simulink model "SignalToNoiseDSKC6713"  (Simulink 6.5)
settings: Solver=FixedStepDiscrete  StartTime=0.0  StopTime=inf  RelTol=1e-3
PreLoadFcn:
  | load dspwlets;
PostLoadFcn:
  | c6000demoscallback
undefined symbols (not defined in the file or in its folder): bit, D, fdesignblkfcn, gcbh
libraries: dspsigops x11, c6713dsklib x4, dspstat3 x3, simulink x1, dspsigattribs x1, dspmathops x1, c6000tgtpreflib x1, dspbioslib x1
CloseFcn:
  | clear fs hid hir lod lor noisdopp ts;
settings Model: RequirementInfo=9  Creator=don  LastModifiedBy=Administrator  CovMetricSettings=d  ExtModeTrigMode=oneshot  ExtModeArmWhenConnect=off  ProdHWDeviceType=TI C6000
settings SolverCC: PositivePriorityOrder=on
settings DataIOCC: LimitDataPoints=off  SaveOutput=off  SaveTime=off  SignalLoggingName=sigsOut
settings OptimizationCC: BlockReduction=off  BooleanDataType=off  InlineParams=on  InlineInvariantSignals=on  RollThreshold=2  OptimizeModelRefInitCode=on  LifeSpan=1  BufferReusableBoundary=off
settings DebuggingCC: CheckExecutionContextPreStartOutputMsg=on  CheckExecutionContextRuntimeOutputMsg=on  SolverPrmCheckMsg=none  InheritedTsInSrcMsg=none  MultiTaskDSMMsg=warning  MultiTaskCondExecSysMsg=none  IntegerOverflowMsg=none  StrictBusMsg=None
settings HardwareCC: ProdBitPerLong=40  ProdIntDivRoundTo=Zero  ProdEndianess=LittleEndian  ProdHWDeviceType=TI C6000  TargetHWDeviceType=32-bit Generic
settings ModelReferenceCC: UpdateModelReferenceTargets=IfOutOfDate
settings RTWCC: SystemTargetFile=ti_c6000_ert.tlc  GenCodeOnly=on  TemplateMakefile=ti_c6000_ert.tmf  ProcessScript=ti_c6000_ert_make_rtw_hook  IncludeERTFirstTime=on
settings CodeAppCC: IgnoreCustomStorageClasses=off  PrefixModelToSubsysFcnNames=off  CustomSymbolStrFcn=$F$N$M
settings C6000ERTTargetCC: TargetFcnLib=ansi_tfl_tmw.mat  GenFloatMathFcnCalls=ANSI_C  UtilityFuncGeneration=Auto  GenerateFullHeader=on  GenerateSampleERTMain=on  GenerateTestInterfaces=off  IsPILTarget=off  ModelReferenceCompliant=off  IncludeMdlTerminateFcn=on  CombineOutputUpdateFcns=on  SuppressErrorStatus=off  IncludeFileDelimiter=Auto  ERTCustomFileBanners=on  SupportAbsoluteTime=on  LogVarNameModifier=rt_  MatFileLogging=off  MultiInstanceERTCode=off  SupportNonFinite=on  SupportComplex=on  PurelyIntegerCode=off  SupportContinuousTime=on  SupportNonInlinedSFcns=on  EnableShiftOperators=on  ParenthesesLevel=Nominal  GenerateErtSFunction=off  GenerateASAP2=off  ExtMode=off  ExtModeTransport=0  ExtModeStaticAlloc=off  ExtModeStaticAllocSize=1000000  ExtModeTesting=off  ExtModeMexFile=ext_comm  InlinedParameterPlacement=NonHierarchical  TargetOS=BareBoardExample  MultiInstanceErrorCode=Error  RateGroupingCode=on  RootIOFormat=Individual arguments  RTWCAPISignals=off  RTWCAPIParams=off  RTWCAPIStates=off  ERTSrcFileBannerTemplate=ert_code_template.cgt  ERTHdrFileBannerTemplate=ert_code_template.cgt  ERTDataSrcFileTemplate=ert_code_template.cgt  ERTDataHdrFileTemplate=ert_code_template.cgt  ERTCustomFileTemplate=example_file_process.tlc  ModuleNamingRule=Unspecified  SignalDisplayLevel=10  ParamTuneLevel=10  GlobalDataDefinition=Auto  DataDefinitionFile=global.c  GlobalDataReference=Auto  DataReferenceFile=global.h  GRTInterface=off  EnableUserReplacementTypes=off  MemSecPackage=--- None ---  MemSecDataConstants=Default  MemSecDataIO=Default  MemSecDataInternal=Default  MemSecDataParameters=Default  MemSecFuncInitTerm=Default  MemSecFuncExecute=Default  exportCCSObj=on  ccsObjName=CCS_Obj  useDSPBIOS=on  ProfileGenCode=off  InlineDSPBlks=on  FPopt=off  memModel=Far_Aggregate  optLevel=Function(-o2)  CompilerVerbosity=Quiet  InterruptThreshOnC6x=off  SymbolicDebugOnC6x=off  RetainAsmFiles=off  RetainObjFiles=on  CreateMapFile=on  UserStackSize=8192  c6000BuildAction=Build_and_execute  OverrunAction=Notify_and_continue  OverrunNotificationMethod=Turn_on_LEDs

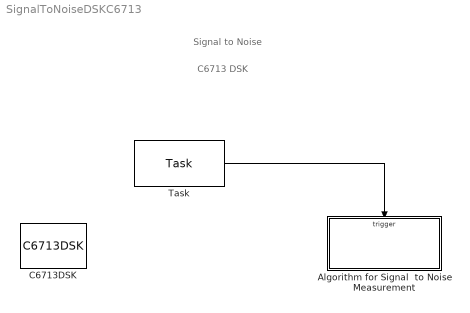
== system SignalToNoiseDSKC6713 ==
  note: C6713 DSK
  note: Signal to Noise
  Algorithm for Signal  to Noise Measurement : Subsystem  TreatAsAtomicUnit=on
  C6713DSK : c6000tgtpreflib/C6713DSK  Tag=C6000 TARGET PREFERENCES BLOCK  SystemSampleTime=-1
  Task : dspbioslib/Task  SystemSampleTime=-1  taskName=Task0  taskPriority=1  taskExecutionOrder=1  taskStackSize=16000  stackMemSegment=IRAM  monitorStackUse=off  taskYield=off  parentmanaget=on  tickres=1/1000  ticklen=32bits  taskTrigger=off
  wires:
  Task/1 -> Algorithm for Signal  to Noise Measurement/Trigger

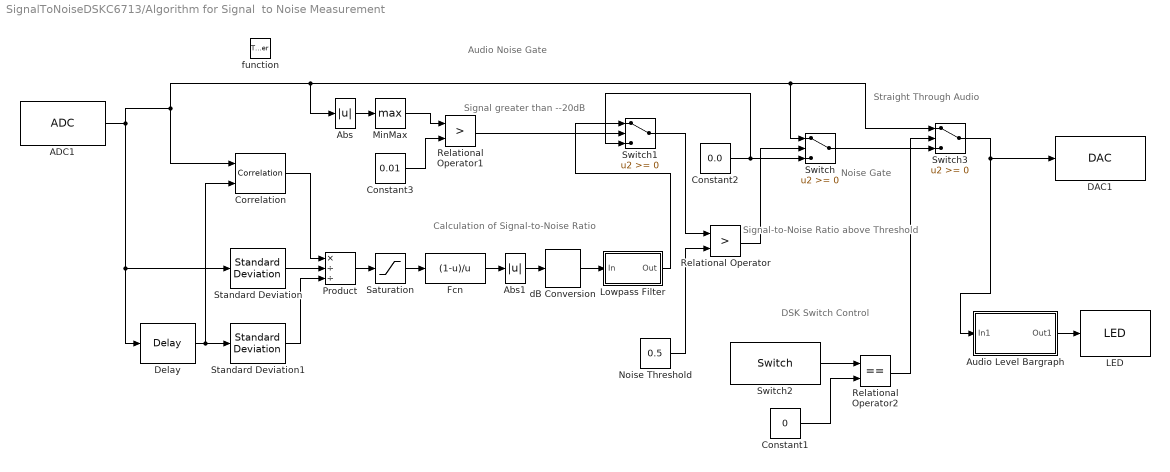
== system SignalToNoiseDSKC6713/Algorithm for Signal  to Noise Measurement ==
  note: Audio Noise Gate
  note: Calculation of Signal-to-Noise Ratio
  note: Signal greater
      |  than --20dB
  note: Straight
      | Through Audio
  note: Noise
      |  Gate
  note: DSK Switch Control
  note: Signal-to-Noise Ratio
      |  above Threshold
  function : TriggerPort  TriggerType=function-call
  ADC1 : c6713dsklib/ADC  ADCsource=Mic In  MicGain=on  Stereo=off  SampleRate=8 kHz  CodecDataFormat=16-bit  OutputDataType=Single  Scaling=Normalize  SourceGain=0.0  FrameSize=128  inheritSampleTime=on
  Abs : Abs  SampleTime=-1  SaturateOnIntegerOverflow=off
  Abs1 : Abs  SampleTime=-1  SaturateOnIntegerOverflow=off
  Audio Level Bargraph : Subsystem
  Constant1 : Constant  Value=0  OutDataType=sfix(16)  ConRadixGroup=Use specified scaling  OutScaling=2^0  SampleTime=inf  FramePeriod=inf
  Constant2 : Constant  Value=0.0  OutDataType=sfix(16)  ConRadixGroup=Use specified scaling  OutScaling=2^0  SampleTime=inf  FramePeriod=inf
  Constant3 : Constant  Value=0.01  OutDataType=sfix(16)  ConRadixGroup=Use specified scaling  OutScaling=2^0  SampleTime=inf  FramePeriod=inf
  Correlation : dspstat3/Correlation  DialogController=dspDDGCreate  DialogControllerArgs=DataTag0  domain=Time  roundingMode=Floor  overflowMode=off
  DAC1 : c6713dsklib/DAC  CodecDataFormat=16-bit  SampleRate=8 kHz  Scaling=Normalize  DacAtten=0.0  OverflowMode=Saturate
  Delay : dspsigops/Delay  dly_unit=Samples  delay=12  ic_detail=off  dif_ic_for_ch=off  dif_ic_for_dly=off  ic=0  reset_popup=None
  Fcn : Fcn  Expr=(1-u)/u
  LED : c6713dsklib/LED
  Lowpass Filter : Subsystem  DialogController=fdesignblkfcn  DialogControllerArgs=DataTag2  InitFcn=fdesignblkfcn(gcbh, {'InitFcn'});
      settings: CopyFcn=fdesignblkfcn(gcbh, {'CopyFcn'});
      mask Type: Lowpass Filter
      mask Description: Design a lowpass filter
      mask Help: helpview(mapfilelocation('dspblks'), 'dsplowpassfilter')
      mask Display: disp('Lowpass')
  MinMax : MinMax  Function=max
  "Noise Threshold " : Constant  Value=0.5  OutDataType=sfix(16)  ConRadixGroup=Use specified scaling  OutScaling=2^0  SampleTime=inf  FramePeriod=inf
  Product : Product  Inputs=*//  RndMeth=Zero
  Relational Operator : RelationalOperator  Operator=>  LogicOutDataTypeMode=Boolean
  Relational Operator1 : RelationalOperator  Operator=>  LogicOutDataTypeMode=Boolean
  Relational Operator2 : RelationalOperator  Operator===  LogicOutDataTypeMode=Boolean
  Saturation : Saturate  UpperLimit=0.99  LowerLimit=-0.99
  Standard Deviation : dspstat3/Standard Deviation  run=off  reset_popup=None
  Standard Deviation1 : dspstat3/Standard Deviation  run=off  reset_popup=None
  Switch : Switch
  Switch1 : Switch
  Switch2 : c6713dsklib/Switch  sw0=on  sw1=on  sw2=on  sw3=on  dType=Integer  Ts=-1
  Switch3 : Switch
  dB Conversion : dspmathops/dB Conversion  SystemSampleTime=-1  dBtype=dB  intype=Power  R=1  fuzz=off
  wires:
  Delay/1 -> Standard Deviation1/1, Correlation/2
  Standard Deviation/1 -> Product/2
  Standard Deviation1/1 -> Product/3
  Product/1 -> Saturation/1
  Saturation/1 -> Fcn/1
  Fcn/1 -> Abs1/1
  "Noise Threshold "/1 -> Relational Operator/2
  Relational Operator/1 -> Switch/2
  Constant2/1 -> Switch/3, Switch1/3
  Audio Level Bargraph/1(Out1) -> LED/1
  ADC1/1 -> Standard Deviation/1, Delay/1, Correlation/1, Abs/1, Switch/1, Switch3/1
  Correlation/1 -> Product/1
  MinMax/1 -> Relational Operator1/1
  Constant3/1 -> Relational Operator1/2
  Relational Operator1/1 -> Switch1/2
  Abs/1 -> MinMax/1
  Abs1/1 -> dB Conversion/1
  dB Conversion/1 -> Lowpass Filter/1(In)
  Switch1/1 -> Relational Operator/1
  Lowpass Filter/1(Out) -> Switch1/1
  Switch2/1 -> Relational Operator2/1
  Constant1/1 -> Relational Operator2/2
  Switch3/1 -> DAC1/1, Audio Level Bargraph/1(In1)
  Switch/1 -> Switch3/3
  Relational Operator2/1 -> Switch3/2

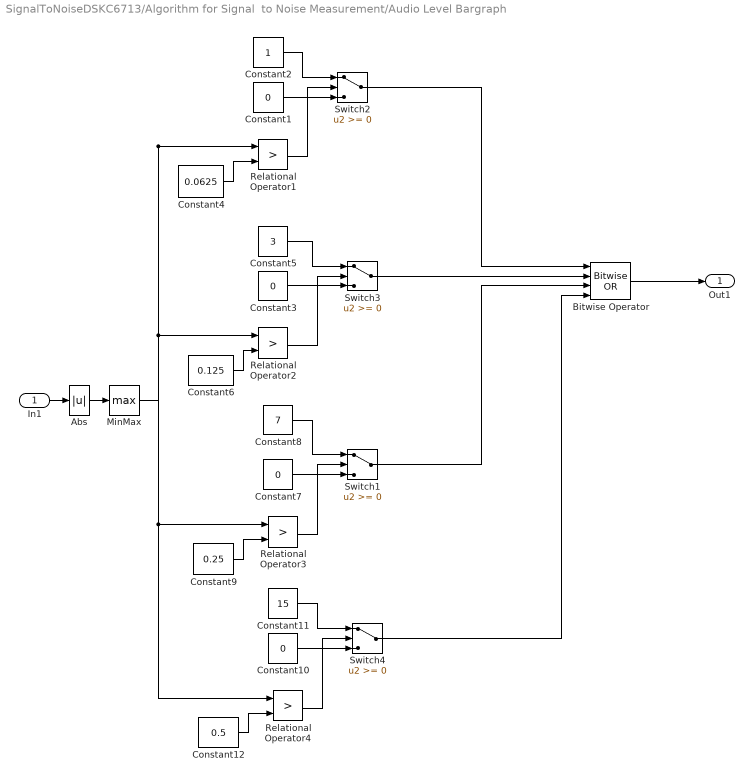
== system SignalToNoiseDSKC6713/Algorithm for Signal  to Noise Measurement/Audio Level Bargraph ==
  In1 : Inport
  Abs : Abs  SampleTime=-1  SaturateOnIntegerOverflow=off
  Bitwise Operator : simulink/Logic and Bit Operations/Bitwise Operator  logicop=OR  UseBitMask=off  NumInputPorts=4  BitMask=bin2dec('11011001')  BitMaskRealWorld=Stored Integer
  Constant{1,3,7,10} (4 alike) : Constant  Value=0  OutDataTypeMode=int8  OutDataType=sfix(16)  ConRadixGroup=Use specified scaling  OutScaling=2^0  SampleTime=inf  FramePeriod=inf
  Constant11 : Constant  Value=15  OutDataTypeMode=int8  OutDataType=sfix(16)  ConRadixGroup=Use specified scaling  OutScaling=2^0  SampleTime=inf  FramePeriod=inf
  Constant12 : Constant  Value=0.5  OutDataType=sfix(16)  ConRadixGroup=Use specified scaling  OutScaling=2^0  SampleTime=inf  FramePeriod=inf
  Constant2 : Constant  Value=1  OutDataTypeMode=int8  OutDataType=sfix(16)  ConRadixGroup=Use specified scaling  OutScaling=2^0  SampleTime=inf  FramePeriod=inf
  Constant4 : Constant  Value=0.0625  OutDataType=sfix(16)  ConRadixGroup=Use specified scaling  OutScaling=2^0  SampleTime=inf  FramePeriod=inf
  Constant5 : Constant  Value=3  OutDataTypeMode=int8  OutDataType=sfix(16)  ConRadixGroup=Use specified scaling  OutScaling=2^0  SampleTime=inf  FramePeriod=inf
  Constant6 : Constant  Value=0.125  OutDataType=sfix(16)  ConRadixGroup=Use specified scaling  OutScaling=2^0  SampleTime=inf  FramePeriod=inf
  Constant8 : Constant  Value=7  OutDataTypeMode=int8  OutDataType=sfix(16)  ConRadixGroup=Use specified scaling  OutScaling=2^0  SampleTime=inf  FramePeriod=inf
  Constant9 : Constant  Value=0.25  OutDataType=sfix(16)  ConRadixGroup=Use specified scaling  OutScaling=2^0  SampleTime=inf  FramePeriod=inf
  MinMax : MinMax  Function=max
  Relational Operator{1..4} (4 alike) : RelationalOperator  Operator=>  LogicOutDataTypeMode=Boolean
  Switch{1..4} (4 alike) : Switch
  Out1 : Outport
  wires:
  In1/1 -> Abs/1
  Bitwise Operator/1 -> Out1/1
  Relational Operator1/1 -> Switch2/2
  Constant4/1 -> Relational Operator1/2
  Constant1/1 -> Switch2/3
  Constant2/1 -> Switch2/1
  Switch2/1 -> Bitwise Operator/1
  Relational Operator2/1 -> Switch3/2
  Constant6/1 -> Relational Operator2/2
  Constant3/1 -> Switch3/3
  Constant5/1 -> Switch3/1
  Switch3/1 -> Bitwise Operator/2
  Relational Operator3/1 -> Switch1/2
  Constant9/1 -> Relational Operator3/2
  Constant7/1 -> Switch1/3
  Constant8/1 -> Switch1/1
  Switch1/1 -> Bitwise Operator/3
  Relational Operator4/1 -> Switch4/2
  Constant12/1 -> Relational Operator4/2
  Constant10/1 -> Switch4/3
  Constant11/1 -> Switch4/1
  Switch4/1 -> Bitwise Operator/4
  Abs/1 -> MinMax/1
  MinMax/1 -> Relational Operator1/1, Relational Operator2/1, Relational Operator3/1, Relational Operator4/1

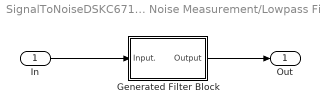
== system SignalToNoiseDSKC6713/Algorithm for Signal  to Noise Measurement/Lowpass Filter ==
  In : Inport
  Generated Filter Block : Subsystem  Tag=FilterWizardSubSystem
      settings: ErrorFcn=dspFilterRealizedInBasicElemsAlgLoopErrFcnCallback
  Out : Outport
  wires:
  In/1 -> Generated Filter Block/1(Input.)
  Generated Filter Block/1(Output) -> Out/1

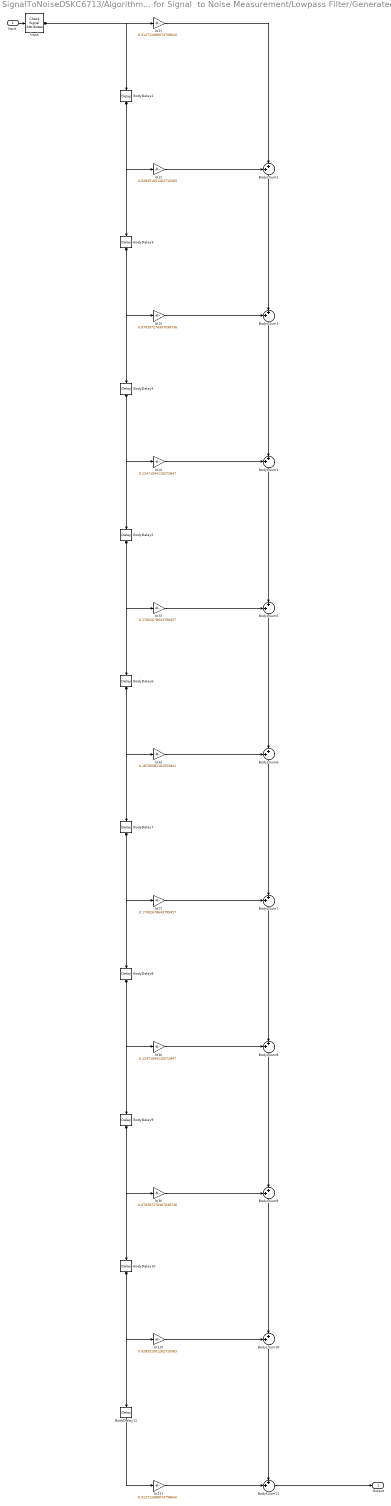
== system SignalToNoiseDSKC6713/Algorithm for Signal  to Noise Measurement/Lowpass Filter/Generated Filter Block ==
  Input. : Inport
  BodyDelay{2..11} (10 alike) : dspsigops/Delay  Orientation=down  dly_unit=Samples  delay=1  ic_detail=off  dif_ic_for_ch=off  dif_ic_for_dly=off  ic=0  reset_popup=None
  BodyLSum{2..10} (9 alike) : Sum  Orientation=down  Inputs=++|  RndMeth=Nearest  SaturateOnIntegerOverflow=on  InputSameDT=on
  BodyLSum11 : Sum  Inputs=++|  RndMeth=Nearest  SaturateOnIntegerOverflow=on  InputSameDT=on
  Input : dspsigattribs/Check Signal Attributes  SystemSampleTime=-1  SigAttribCheckMethod=Matches attributes exactly  Complexity=Ignore  Frame=Ignore  DimsCheckMethod=Ignore  Dimensions=1-D  DatatypeCheckMethod=Is not...  DatatypeGeneral=Floating-point  DtypeFloatSpecific=Any floating-point  DtypeFixedSpecific=Any fixed-point  DtypeIntSpecific=Any integer  SampleMode=Ignore
  b(1) : Gain  Gain=0.012711089073758642  SaturateOnIntegerOverflow=on
  b(10) : Gain  Gain=0.028351001262710365  SaturateOnIntegerOverflow=on
  b(11) : Gain  Gain=0.012711089073758642  SaturateOnIntegerOverflow=on
  b(2) : Gain  Gain=0.028351001262710365  SaturateOnIntegerOverflow=on
  b(3) : Gain  Gain=0.070397276307038736  SaturateOnIntegerOverflow=on
  b(4) : Gain  Gain=0.12471094110572847  SaturateOnIntegerOverflow=on
  b(5) : Gain  Gain=0.17002678643799457  SaturateOnIntegerOverflow=on
  b(6) : Gain  Gain=0.18760581162553841  SaturateOnIntegerOverflow=on
  b(7) : Gain  Gain=0.17002678643799457  SaturateOnIntegerOverflow=on
  b(8) : Gain  Gain=0.12471094110572847  SaturateOnIntegerOverflow=on
  b(9) : Gain  Gain=0.070397276307038736  SaturateOnIntegerOverflow=on
  Output : Outport
  wires:
  Input./1 -> Input/1
  Input/1 -> b(1)/1, BodyDelay2/1
  b(1)/1 -> BodyLSum2/2
  BodyDelay2/1 -> b(2)/1, BodyDelay3/1
  b(2)/1 -> BodyLSum2/1
  BodyLSum2/1 -> BodyLSum3/2
  BodyDelay3/1 -> b(3)/1, BodyDelay4/1
  b(3)/1 -> BodyLSum3/1
  BodyLSum3/1 -> BodyLSum4/2
  BodyDelay4/1 -> b(4)/1, BodyDelay5/1
  b(4)/1 -> BodyLSum4/1
  BodyLSum4/1 -> BodyLSum5/2
  BodyDelay5/1 -> b(5)/1, BodyDelay6/1
  b(5)/1 -> BodyLSum5/1
  BodyLSum5/1 -> BodyLSum6/2
  BodyDelay6/1 -> b(6)/1, BodyDelay7/1
  b(6)/1 -> BodyLSum6/1
  BodyLSum6/1 -> BodyLSum7/2
  BodyDelay7/1 -> b(7)/1, BodyDelay8/1
  b(7)/1 -> BodyLSum7/1
  BodyLSum7/1 -> BodyLSum8/2
  BodyDelay8/1 -> b(8)/1, BodyDelay9/1
  b(8)/1 -> BodyLSum8/1
  BodyLSum8/1 -> BodyLSum9/2
  BodyDelay9/1 -> b(9)/1, BodyDelay10/1
  b(9)/1 -> BodyLSum9/1
  BodyLSum9/1 -> BodyLSum10/2
  BodyDelay10/1 -> b(10)/1, BodyDelay11/1
  b(10)/1 -> BodyLSum10/1
  BodyLSum10/1 -> BodyLSum11/1
  BodyDelay11/1 -> b(11)/1
  b(11)/1 -> BodyLSum11/2
  BodyLSum11/1 -> Output/1
